simulink model "Motorlab_PWM"  (R2019a)
settings: Solver=FixedStepDiscrete  StartTime=0.0  StopTime=10.0  FixedStep=0.0001  RelTol=1e-3
undefined symbols (not defined in the file): Simulink_STM32F4_Discovery
libraries: GPIO_Lib x2, TIMERS_Lib x2, USART_Lib x2, simulink x1, STM32_Config_Lib x1
settings Model: Creator=alexkim92  LastModifiedBy=alexk
settings OptimizationCC: DefaultParameterBehavior=Inlined  EnhancedBackFolding=on  PassReuseOutputArgsAs=Individual arguments  OptimizeBlockOrder=speed  DifferentSizesBufferReuse=on  OptimizationCustomize=off
settings DebuggingCC: ParameterTunabilityLossMsg=error
settings HardwareCC: ProdBitPerPointer=32  ProdBitPerSizeT=32  ProdBitPerPtrDiffT=32  ProdLargestAtomicInteger=Long  ProdWordSize=32  ProdHWDeviceType=STM32CortexM
settings SFSimCC: MATLABDynamicMemAlloc=off
settings RTWCC: SystemTargetFile=stm32.tlc  TemplateMakefile=stm32.tmf  Description=stm32 (Embedded Target)  GenerateReport=on  IncludeHyperlinkInReport=on  GenerateTraceInfo=on  GenerateTraceReport=on  GenerateTraceReportSl=on  GenerateTraceReportSf=on  GenerateTraceReportEml=on
settings CodeAppCC: ForceParamTrailComments=on  IgnoreCustomStorageClasses=off  MaxIdLength=64  OperatorAnnotations=on  SimulinkDataObjDesc=on  SFDataObjDesc=on  CustomSymbolStrType=$N$R$M  SimulinkBlockComments=off
settings STFCustomTargetCC: CodeReplacementLibrary=ARM CMSIS SIN COS  MultiwordLength=256  ParMdlRefBuildCompliant=on  IncludeMdlTerminateFcn=off  CombineOutputUpdateFcns=on  ERTCustomFileBanners=on  SupportContinuousTime=off  SupportNonInlinedSFcns=off  RemoveResetFunc=on  MATLABClassNameForMDSCustomization=Simulink.SoftwareTarget.ERTCustomization  GRTInterface=off  SystemTargetFile=stm32.tlc
settings ERTTargetCC: CodeReplacementLibrary=ARM CMSIS SIN COS  CompOptLevelCompliant=off  ConcurrentExecutionCompliant=off  IncludeMdlTerminateFcn=off  ModelStepFunctionPrototypeControlCompliant=off  CPPClassGenCompliant=off  UseToolchainInfoCompliant=off  ExtModeStaticAllocSize=256  ExtModeMexArgs=0,1,115200,10  InlinedParameterPlacement=NonHierarchical  ERTSrcFileBannerTemplate=sourceFileTemplate.cgt  ERTHdrFileBannerTemplate=sourceFileTemplate.cgt  ERTDataSrcFileTemplate=sourceFileTemplate.cgt  ERTDataHdrFileTemplate=sourceFileTemplate.cgt  ERTCustomFileTemplate=customRoutineProcess.tlc

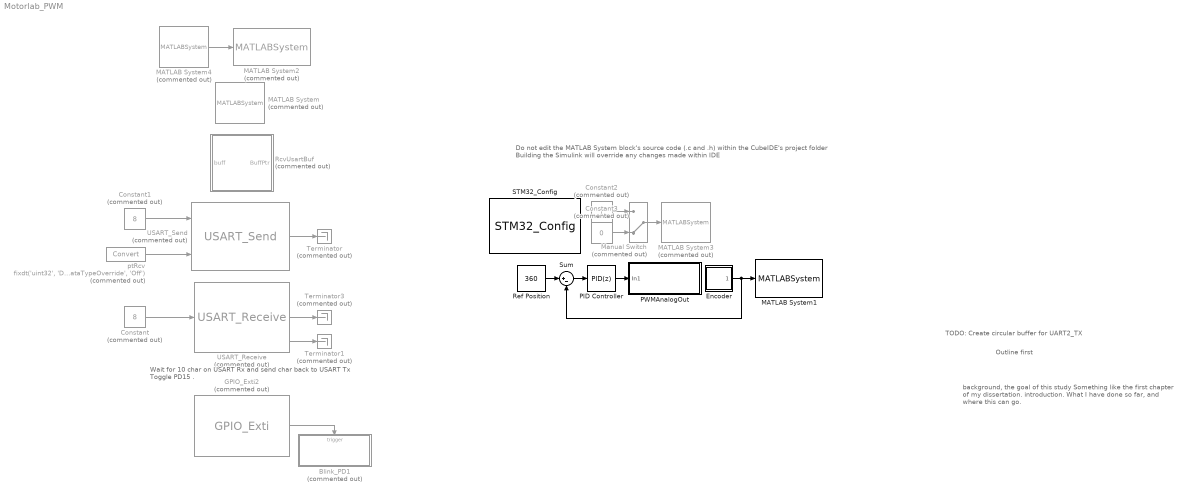
== system Motorlab_PWM ==
  note: Outline first
  note: background, the goal of this study
      | Something like the first chapter of my dissertation. introduction.
      | What I have done so far, and where this can go.
  note: TODO: Create circular buffer for UART2_TX
  note: Do not edit the MATLAB System block's source code (.c and .h) within the CubeIDE's project folder
      | Building the Simulink will override any changes made within IDE
  note: Wait for 10 char on USART Rx and send char back to USART Tx
      | Toggle PD15 .
  Blink_PD1 : Subsystem  Commented=on  TreatAsAtomicUnit=on
  Constant : Constant  Commented=on  Value=8
  Constant1 : Constant  Commented=on  Value=8
  Constant2 : Constant  Commented=on  SampleTime=-1
  Constant3 : Constant  Commented=on  Value=0  SampleTime=-1
  Encoder : Subsystem
  GPIO_Exti2 : GPIO_Lib/GPIO_Exti  Commented=on  Port_name=GPIOA  Pin_0=on  Pin_1=off  Pin_2=off  Pin_3=off  Pin_4=off  Pin_5=off  Pin_6=off  Pin_7=off  Pin_8=off  Pin_9=off  Pin_10=off  Pin_11=off  Pin_12=off  Pin_13=off  Pin_14=off  Pin_15=off  PinList=GPIOA0
      settings: SourceProductName=Target Support Package - STM32 Adapter
  MATLAB System : MATLABSystem  Commented=on  System=Encoder  SampleTime=-1
      mask Type: Encoder
      mask Display:
      | disp('Encoder');
      | port_label('output',1,'y');
  MATLAB System1 : MATLABSystem  Priority=16  System=UART2_TX
      mask Type: UART2_TX
      mask Display:
      | disp('UART2_TX');
      | port_label('input',1,'u');
  MATLAB System2 : MATLABSystem  Commented=on  System=PWMAnalogOut
      mask Type: PWMAnalogOut
      mask Display:
      | disp('PWM Analog Out');
      | port_label('input',1,'u');
  MATLAB System3 : MATLABSystem  Priority=-1  Commented=on  System=DigitalOut
      mask Type: DigitalOut
      mask Display:
      | disp('DigitalOut');
      | port_label('input',1,'u');
  MATLAB System4 : MATLABSystem  Commented=on  System=PIDController  P=0.1  I=0.0  D=0.0  IntegralLim=1.0  DT=0.001  OutLim=3.0
      mask Type: PIDController
      mask Display:
      | disp('PID');
      | port_label('input',1,'u');
      | port_label('output',1,'y');
  Manual Switch : ManualSwitch  Commented=on  CurrentSetting=0
  PID Controller : simulink/Continuous/PID Controller  Controller=PID  Form=Parallel  TimeDomain=Discrete-time  SampleTime=-1  IntegratorMethod=Forward Euler  FilterMethod=Forward Euler  ControllerParametersSource=internal  P=0.1  I=0  D=0.001  UseFilter=on  N=100  TunerSelectOption=Transfer Function Based (PID Tuner App)  InitialConditionSource=internal  InitialConditionForIntegrator=0  InitialConditionForFilter=0  DifferentiatorICPrevScaledInput=0  ExternalReset=none  TrackingMode=off  Kt=1  LimitOutput=off  UpperSaturationLimit=inf  LowerSaturationLimit=-inf  LinearizeAsGain=on  AntiWindupMode=none  Kb=1  PGainOutDataTypeStr=double  PProdOutDataTypeStr=double  POutMin=[]  POutMax=[]  IOutMin=[]  IOutMax=[]  DGainOutDataTypeStr=double  DProdOutDataTypeStr=double  DOutMin=[]  DOutMax=[]  NGainOutDataTypeStr=double  NProdOutDataTypeStr=double  NOutMin=[]  NOutMax=[]  SumOutDataTypeStr=double  SumOutMin=[]  SumOutMax=[]  SaturationOutMin=[]  SaturationOutMax=[]  PParamMin=[]  PParamMax=[]  IParamMin=[]  IParamMax=[]  DParamMin=[]  DParamMax=[]  NParamMin=[]  NParamMax=[]  KbParamMin=[]  KbParamMax=[]  KtParamMin=[]  KtParamMax=[]  KbOutMin=[]  KbOutMax=[]  KtOutMin=[]  KtOutMax=[]  IntegratorOutMin=[]  IntegratorOutMax=[]  FilterOutMin=[]  FilterOutMax=[]  SumI1OutMin=[]  SumI1OutMax=[]  SumI2OutMin=[]  SumI2OutMax=[]  SumI3OutMin=[]  SumI3OutMax=[]  SumI4OutMin=[]  SumI4OutMax=[]  SumDOutMin=[]  SumDOutMax=[]  DifferentiatorOutMin=[]  DifferentiatorOutMax=[]  FilterDiffOutCoefMin=[]  FilterDiffOutCoefMax=[]  ReciprocalOutMin=[]  ReciprocalOutMax=[]  SumDenOutMin=[]  SumDenOutMax=[]  SumNumOutMin=[]  SumNumOutMax=[]  DivideOutMin=[]  DivideOutMax=[]  IntegratorContinuousStateAttributes=''  IntegratorStateMustResolveToSignalObject=off  IntegratorRTWStateStorageClass=Auto  FilterContinuousStateAttributes=''  FilterStateMustResolveToSignalObject=off  FilterRTWStateStorageClass=Auto  ParallelPVariant=InternalParameters  IdealPVariant=Disabled  IVariant=InternalParameters  DVariant=InternalParameters  IntegratorVariant=Discrete  SatVariant=Disabled  AWVariant=Passthrough  PCopyVariant=Disabled  TRVariant=Disabled  FdbkBlocksVariant=Forward  IdealPFdbkVariant=Disabled  SatFdbkVariant=Disabled  DerivativeFilterVariant=ForwardEulerFilter  NVariant=InternalParameters  NCopyVariant=Disabled  FilterICVariant=InternalICsFilter  IntegratorICVariant=InternalICs  ExternalResetVariant=Disabled  TRSumVariant=Passthrough  SumFdbkVariant=Disabled  SumVariant=Sum_PID
  PWMAnalogOut : Subsystem
  RcvUsartBuf : MATLAB Function  Commented=on  TreatAsAtomicUnit=on
  Ref Position : Constant  Value=360  SampleTime=-1
  STM32_Config : STM32_Config_Lib/STM32_Config  Priority=0  Project_Path=.\..\Simulink_STM32F4_Discovery\  Config_File=Simulink_STM32F4_Discovery.ioc  MCU_Name=STM32F407VGTx
      settings: SourceProductName=Target Support Package - STM32 Adapter
  Sum : Sum  Inputs=|+-
  Terminator : Terminator  Commented=on
  Terminator1 : Terminator  Commented=on
  Terminator3 : Terminator  Commented=on
  USART_Receive : USART_Lib/USART_Receive  Commented=on  USART_name=USART2  Buff_size=32  nbUsart=1  Soft_it=on  Soft_num=0  usartMode=Asynchronous  usartDma_Rx=off  usartDma_Tx=on  usartIt=on
      settings: SourceProductName=Target Support Package - STM32 Adapter
  USART_Send : USART_Lib/USART_Send  Commented=on  USART_name=USART2  Buff_size=32  nbUsart=1  usartMode=Asynchronous  usartDma_Rx=off  usartDma_Tx=on  usartIt=on
      settings: SourceProductName=Target Support Package - STM32 Adapter
  ptRcv : DataTypeConversion  Commented=on  OutDataTypeStr=fixdt('uint32', 'DataTypeOverride', 'Off')
  wires:
  USART_Send/1 -> Terminator/1
  GPIO_Exti2/1 -> Blink_PD1/Trigger
  Constant/1 -> USART_Receive/1
  USART_Receive/3 -> Terminator1/1
  USART_Receive/2 -> Terminator3/1
  Constant1/1 -> USART_Send/1
  ptRcv/1 -> USART_Send/2
  Constant2/1 -> Manual Switch/1
  Constant3/1 -> Manual Switch/2
  Ref Position/1 -> Sum/1
  MATLAB System4/1 -> MATLAB System2/1
  Sum/1 -> PID Controller/1
  PID Controller/1 -> PWMAnalogOut/1(In1)
  Encoder/1(Out1) -> Sum/2, MATLAB System1/1
  Manual Switch/1 -> MATLAB System3/1

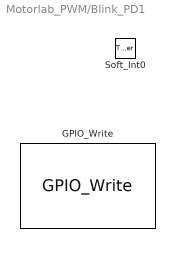
== system Motorlab_PWM/Blink_PD1 ==
  Soft_Int0 : TriggerPort  TriggerType=function-call  VariantControl=Variant
  GPIO_Write : GPIO_Lib/GPIO_Write  Port_name=GPIOD  Pin0=off  Toggle_Pin0=off  Pin1=off  Toggle_Pin1=off  Pin2=off  Toggle_Pin2=off  Pin3=off  Toggle_Pin3=off  Pin4=off  Toggle_Pin4=off  Pin5=off  Toggle_Pin5=off  Pin6=off  Toggle_Pin6=off  Pin7=off  Toggle_Pin7=off  Pin8=off  Toggle_Pin8=off  Pin9=off  Toggle_Pin9=off  Pin10=off  Toggle_Pin10=off  Pin11=off  Toggle_Pin11=off  Pin12=on  Toggle_Pin12=on  Pin13=on  Toggle_Pin13=on  Pin14=on  Toggle_Pin14=on  Pin15=on  Toggle_Pin15=on  PinList="GPIOB11GPIOC0GPIOD12  13  14  15"
      settings: SourceProductName=Target Support Package - STM32 Adapter

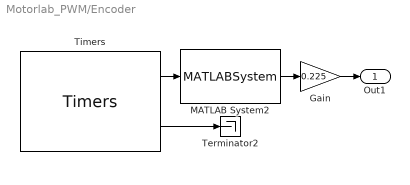
== system Motorlab_PWM/Encoder ==
  Gain : Gain  Gain=0.225  OutDataTypeStr=double
  MATLAB System2 : MATLABSystem  System=Count2Angle
      mask Type: Count2Angle
      mask Display:
      | disp('Count2Angle');
      | port_label('input',1,'u');
      | port_label('output',1,'y');
  Terminator2 : Terminator
  Timers : TIMERS_Lib/Timers  currentTIM=TIM1  TIM_Name=TIM1  sysUsingTimer=on  TIM_APBClock=168000000  TIM_Set_Clk=off  TIM_Prescaler=0  TIM_Clock=168000000.00  Variable_frequency=off  TIM_Set_OutFreq=off  TIM_ARR=65536  Output_frequency=2563.48  Repetition_counter=0  TIM_Mode=Up  TIM_DMA=none  TIM_IRQ=off  TIM_IRQ_ONLY=off  TIM_UP=off  TIM_TRG=off  TIM_COM=off  TIM_BRK=off  NbTIM=2  CH1_enable=on  CH1N_enable=off  CH1_type=Input_Encoder  CH1_DMA=off  CH1_int=off  CH1_edge=Rising  CH1_div=1  CH1_variable_duty=off  CH1_set_pulse=off  CH1_output_duty=0.00  CH1_pulse=0  CH2_enable=on  CH2N_enable=off  CH2_type=Input_Encoder  CH2_DMA=off  CH2_int=off  CH2_edge=Rising  CH2_div=1  CH2_variable_duty=off  CH2_set_pulse=off  CH2_output_duty=0.00  CH2_pulse=0  CH3_enable=off  CH3N_enable=off  CH3_type=Unknown  CH3_DMA=off  CH3_int=off  CH3_edge=Rising  CH3_div=1  CH3_variable_duty=off  CH3_set_pulse=off  CH3_output_duty=0.00  CH3_pulse=0  CH4_enable=off  CH4N_enable=off  CH4_type=Unknown  CH4_DMA=off  CH4_int=off  CH4_edge=Rising  CH4_div=1  CH4_variable_duty=off  CH4_set_pulse=off  CH4_output_duty=0.00  CH4_pulse=0
      settings: SourceProductName=Target Support Package - STM32 Adapter
  Out1 : Outport
  wires:
  MATLAB System2/1 -> Gain/1
  Gain/1 -> Out1/1
  Timers/1 -> MATLAB System2/1
  Timers/2 -> Terminator2/1

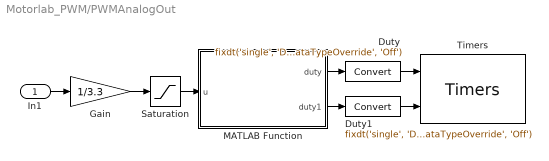
== system Motorlab_PWM/PWMAnalogOut ==
  In1 : Inport
  Duty : DataTypeConversion  OutDataTypeStr=fixdt('single', 'DataTypeOverride', 'Off')
  Duty1 : DataTypeConversion  OutDataTypeStr=fixdt('single', 'DataTypeOverride', 'Off')
  Gain : Gain  Gain=1/3.3
  MATLAB Function : MATLAB Function  TreatAsAtomicUnit=on
  Saturation : Saturate  UpperLimit=1  LowerLimit=-1
  Timers : TIMERS_Lib/Timers  currentTIM=TIM3  TIM_Name=TIM3  sysUsingTimer=on  TIM_APBClock=84000000  TIM_Set_Clk=off  TIM_Prescaler=2  TIM_Clock=28000000.00  Variable_frequency=off  TIM_Set_OutFreq=off  TIM_ARR=140  Output_frequency=200000.00  Repetition_counter=0  TIM_Mode=Up  TIM_DMA=none  TIM_IRQ=off  TIM_IRQ_ONLY=off  TIM_UP=off  TIM_TRG=off  TIM_COM=off  TIM_BRK=off  NbTIM=2  CH1_enable=on  CH1N_enable=off  CH1_type=Output_PWM  CH1_DMA=off  CH1_int=off  CH1_edge=Rising  CH1_div=1  CH1_variable_duty=on  CH1_set_pulse=off  CH1_output_duty=0.00  CH1_pulse=0  CH2_enable=on  CH2N_enable=off  CH2_type=Output_PWM  CH2_DMA=off  CH2_int=off  CH2_edge=Rising  CH2_div=1  CH2_variable_duty=on  CH2_set_pulse=off  CH2_output_duty=0.00  CH2_pulse=0  CH3_enable=off  CH3N_enable=off  CH3_type=Unknown  CH3_DMA=off  CH3_int=off  CH3_edge=Rising  CH3_div=1  CH3_variable_duty=off  CH3_set_pulse=off  CH3_output_duty=0.00  CH3_pulse=0  CH4_enable=off  CH4N_enable=off  CH4_type=Unknown  CH4_DMA=off  CH4_int=off  CH4_edge=Rising  CH4_div=1  CH4_variable_duty=off  CH4_set_pulse=off  CH4_output_duty=0.00  CH4_pulse=0
      settings: SourceProductName=Target Support Package - STM32 Adapter
  wires:
  In1/1 -> Gain/1
  Saturation/1 -> MATLAB Function/1(u)
  Gain/1 -> Saturation/1
  Duty1/1 -> Timers/2
  MATLAB Function/1(duty) -> Duty/1
  MATLAB Function/2(duty1) -> Duty1/1
  Duty/1 -> Timers/1

== matlab function Motorlab_PWM/PWMAnalogOut/MATLAB Function ==
  data: u input; duty output; duty1 output
function [duty, duty1] = dutyCycle(u)

duty  = double(u);
duty1 = duty;
% duty = ((duty+1)/2)*double(100); %Add 1 to go from -1;1 to 0;2 so /2 and must give percentage
% duty1 = ((duty1+1)/2)*double(100); %Add 1 to go from -1;1 to 0;2 so /2 and must give percentage
if (duty < 0)
    duty  = double(0);
    duty1 = -double(u)*100;
else
    duty  = double(u)*100;
    duty1 = double(0);
end
end

== matlab function Motorlab_PWM/RcvUsartBuf ==
  data: BuffPtr output uint32 size=1; buff input
function BuffPtr = convert(buff)
if coder.target('Sfun')
    % Executing in MATLAB, Buff is null
    BuffPtr = uint32(0);
    %NbChar = uint16(0);
else
    coder.cinclude('getBuffPtr.h');
    % Executing in the generated code.
    BuffPtr = coder.ceval('getBuffPtr',coder.rref(buff));
end
end
